simulink model "BeatDetector"  (R2012b)
settings: Solver=FixedStepDiscrete  StartTime=0.0  StopTime=50  RelTol=1e-3
PreLoadFcn:
  | % load model data
  | BeatDetectorData
values from neighbouring files (symbols this model uses):
  T1 = Simulink.Parameter    [BeatDetectorData.m]
  T2 = Simulink.Parameter    [BeatDetectorData.m]
  T4 = Simulink.Parameter    [BeatDetectorData.m]
  T5 = Simulink.Parameter    [BeatDetectorData.m]
settings Model: Creator=aanantha  LastModifiedBy=klindqvi
settings DataIOCC: SaveFormat=Structure  SignalLoggingSaveFormat=ModelDataLogs  SaveOutput=off  SaveTime=off  SignalLoggingName=logsOut
settings OptimizationCC: InlineParams=on  OptimizeModelRefInitCode=on  LifeSpan=1
settings DebuggingCC: ReadBeforeWriteMsg=DisableAll  WriteAfterWriteMsg=DisableAll  WriteAfterReadMsg=DisableAll  SolverPrmCheckMsg=none  InheritedTsInSrcMsg=none  ParameterPrecisionLossMsg=none  FcnCallInpInsideContextMsg=EnableAllAsWarning
settings HardwareCC: ProdLargestAtomicInteger=Long  ProdLargestAtomicFloat=Double  ProdEndianess=LittleEndian  ProdHWDeviceType=ARM Compatible->ARM Cortex
settings ModelReferenceCC: ModelReferenceNumInstancesAllowed=Single
settings RTWCC: SystemTargetFile=ert.tlc  TemplateMakefile=ert_default_tmf  Description=Embedded Coder  GenerateReport=on  RTWVerbose=off  ProcessScript=ert_make_rtw_hook  IncludeHyperlinkInReport=on  LaunchReport=on  PortableWordSizes=on  CodeProfilingSaveOptions=AllData  GenerateTraceInfo=on  GenerateTraceReportSl=on  GenerateTraceReportSf=on  GenerateTraceReportEml=on  GenerateCodeMetricsReport=on
settings CodeAppCC: IgnoreCustomStorageClasses=off
settings ERTTargetCC: CodeReplacementLibrary=GCC ARM Cortex-A8  MultiwordLength=2048  GenerateSampleERTMain=on  ERTCustomFileTemplate=example_file_process.tlc  ConvertIfToSwitch=off  SuppressUnreachableDefaultCases=off

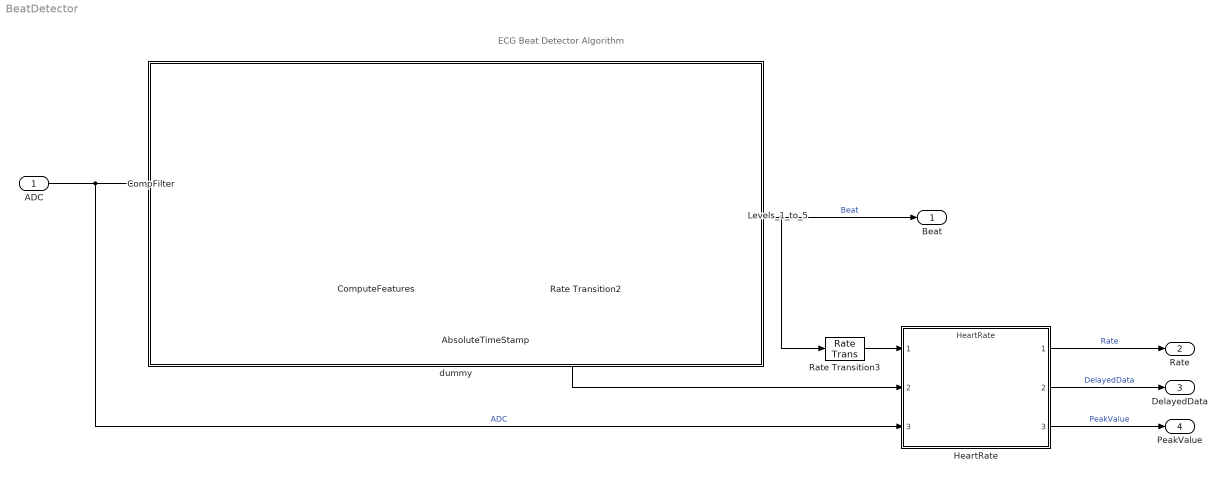
== system BeatDetector ==
  note: ECG Beat Detector Algorithm
  ADC : Inport  RequirementInfo={} %GIDa_ae15db4f_64d4_4e3e_b306_217f7810fee7  OutDataTypeStr=single  PortDimensions=1  SampleTime=[0.001,0]
  AbsoluteTimeStamp : ModelReference  RequirementInfo={} %GIDa_4fcaf68c_811c_40b7_b73f_aee2f921e51d  ModelNameDialog=AbsTimeStamp  SimulationMode=Normal  ModelReferenceVersion=1.244  CopyOfModelName=AbsTimeStamp  DefaultDataLogging=on
  CompFilter : ModelReference  ModelNameDialog=CompFilter  SimulationMode=Normal  ModelReferenceVersion=1.286  CopyOfModelName=CompFilter  DefaultDataLogging=on
  ComputeFeatures : ModelReference  RequirementInfo={} %GIDa_0d581a75_6987_4f24_b98b_7c580a85a396  ModelNameDialog=CompFeatures  SimulationMode=Normal  ModelReferenceVersion=1.282  CopyOfModelName=CompFeatures  DefaultDataLogging=on
  HeartRate : ModelReference  ModelNameDialog=HeartRate  SimulationMode=Normal  ModelReferenceVersion=1.260  CopyOfModelName=HeartRate  DefaultDataLogging=on
  Levels_1_to_5 : Subsystem  RequirementInfo={} %GIDa_bdac3012_1be4_4ef4_889a_c9ca22c44ead
  Rate Transition2 : RateTransition  Deterministic=off
  Rate Transition3 : RateTransition  Deterministic=off  OutPortSampleTime=.001
  dummy : Subsystem  mask{BuffSize=300}
      mask prompts: BuffSize "Buffer Size"
      mask Display: disp('')
  Beat : Outport  RequirementInfo={} %GIDa_cbcaf2f7_287a_43b5_9f3b_34ec9f1a93af  OutDataTypeStr=boolean  PortDimensions=1  SampleTime=[0.08900000000000001,0]
  Rate : Outport  RequirementInfo={} %GIDa_f8020fb5_5ba9_4733_a033_bc7a96b53302  Port=2  OutDataTypeStr=double  PortDimensions=1  SampleTime=[0.001,0]
  DelayedData : Outport  RequirementInfo={} %GIDa_22e24252_a14a_49ee_bd7a_33c06ddc0959  Port=3  OutDataTypeStr=single  PortDimensions=1  SampleTime=[0.001,0]
  PeakValue : Outport  RequirementInfo={} %GIDa_58320da4_9ae1_41e7_bbcb_5dafbfce478b  Port=4  OutDataTypeStr=double  PortDimensions=1  SampleTime=[0.001,0]
  wires:
  AbsoluteTimeStamp/1 -> HeartRate/2, Rate Transition2/1
  Rate Transition2/1 -> Levels_1_to_5/4(time)
  ComputeFeatures/3 -> Levels_1_to_5/3(Feature3)
  ComputeFeatures/2 -> Levels_1_to_5/2(Feature2)
  ComputeFeatures/1 -> Levels_1_to_5/1(Feature1)
  ADC/1 -> HeartRate/3, CompFilter/1  "ADC"
  HeartRate/1 -> Rate/1  "Rate"
  Rate Transition3/1 -> HeartRate/1
  Levels_1_to_5/1(Beat) -> Rate Transition3/1, Beat/1  "Beat"
  HeartRate/2 -> DelayedData/1  "DelayedData"
  HeartRate/3 -> PeakValue/1  "PeakValue"
  CompFilter/1 -> ComputeFeatures/1

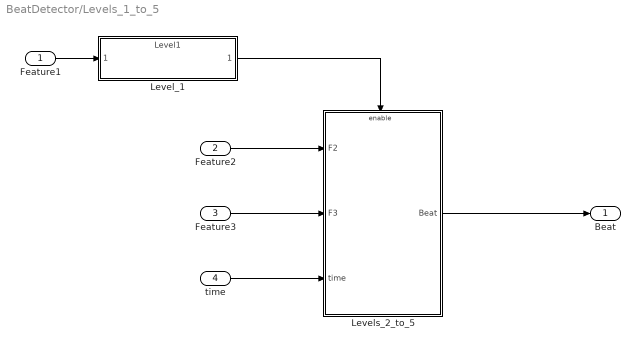
== system BeatDetector/Levels_1_to_5 ==
  Feature1 : Inport
  Feature2 : Inport  Port=2
  Feature3 : Inport  Port=3
  time : Inport  Port=4
  Level_1 : ModelReference  RequirementInfo={} %GIDa_ecf15834_5fdb_4143_ac3d_f4c16752f013  ModelNameDialog=Level1  SimulationMode=Normal  ModelReferenceVersion=1.249  CopyOfModelName=Level1  DefaultDataLogging=on
  Levels_2_to_5 : Subsystem  RequirementInfo={} %GIDa_1cf805d4_ef6b_4316_a489_e2f5af0c56ed
  Beat : Outport
  wires:
  Feature3/1 -> Levels_2_to_5/2(F3)
  Feature2/1 -> Levels_2_to_5/1(F2)
  time/1 -> Levels_2_to_5/3(time)
  Levels_2_to_5/1(Beat) -> Beat/1
  Feature1/1 -> Level_1/1
  Level_1/1 -> Levels_2_to_5/Enable

== system BeatDetector/dummy ==

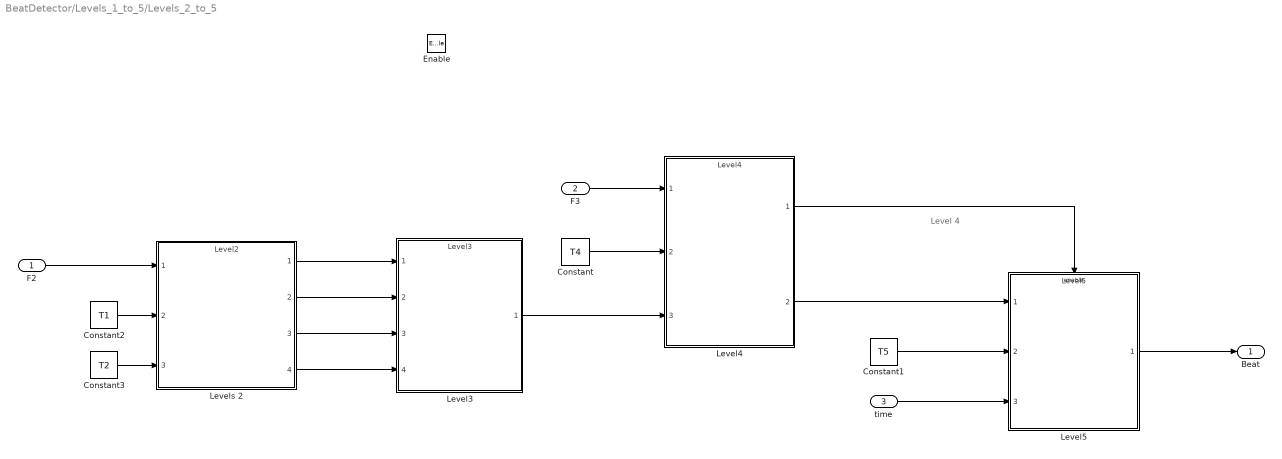
== system BeatDetector/Levels_1_to_5/Levels_2_to_5 ==
  note: Level 4
  F2 : Inport
  F3 : Inport  Port=2
  time : Inport  Port=3
  Enable : EnablePort
  Constant : Constant  RequirementInfo={} %GIDa_7a390ae0_4b96_4b0c_a3a5_8f47fe2d71f3  Value=T4
  Constant1 : Constant  RequirementInfo={} %GIDa_97bae892_9452_4f30_9ccb_ccfaa9bac484  Value=T5
  Constant2 : Constant  RequirementInfo={} %GIDa_1f1e42ec_f1a7_4d34_98d2_f4597468064b  Value=T1
  Constant3 : Constant  RequirementInfo={} %GIDa_7a9dcc6c_b92e_44d1_9b6b_de41eaa0bf68  Value=T2
  Level3 : ModelReference  ModelNameDialog=Level3  SimulationMode=Normal  ModelReferenceVersion=1.249  CopyOfModelName=Level3  DefaultDataLogging=on
  Level4 : ModelReference  ModelNameDialog=Level4  SimulationMode=Normal  ModelReferenceVersion=1.249  CopyOfModelName=Level4  DefaultDataLogging=on
  Level5 : ModelReference  RequirementInfo={} %GIDa_d159189b_af90_4e61_9edb_b9319665060f  ModelNameDialog=Level5  SimulationMode=Normal  ModelReferenceVersion=1.248  CopyOfModelName=Level5  DefaultDataLogging=on  EnablePortName=Enable  EnablePortStatesWhenEnabling=held
  Levels 2 : ModelReference  ModelNameDialog=Level2  SimulationMode=Normal  ModelReferenceVersion=1.252  CopyOfModelName=Level2  DefaultDataLogging=on
  Beat : Outport  RequirementInfo={} %GIDa_2557b2d8_8f9d_4b05_8e6e_ab92a46b1d03  OutputWhenDisabled=reset  InitialOutput=false
  wires:
  time/1 -> Level5/3
  Level5/1 -> Beat/1
  Constant1/1 -> Level5/2
  Constant3/1 -> Levels 2/3
  Constant2/1 -> Levels 2/2
  F2/1 -> Levels 2/1
  Levels 2/1 -> Level3/1
  Levels 2/2 -> Level3/2
  Levels 2/3 -> Level3/3
  Levels 2/4 -> Level3/4
  F3/1 -> Level4/1
  Constant/1 -> Level4/2
  Level3/1 -> Level4/3
  Level4/1 -> Level5/Enable
  Level4/2 -> Level5/1
